simulink model "ster_cyfrowe"  (R2021b)
settings: Solver=VariableStepAuto  StartTime=0.0  StopTime=""  RelTol=1e-3
undefined symbols (not defined in the file or in its folder): kr, Td, Ti, Tp
settings Model: Creator=roman  LastModifiedBy=roman

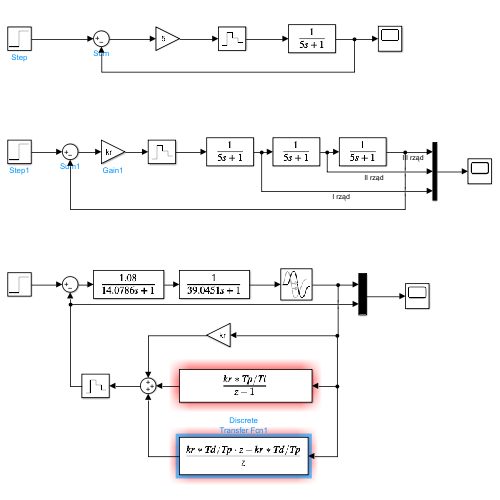
[thumbnail: Simulink's stored preview of the top-level diagram]
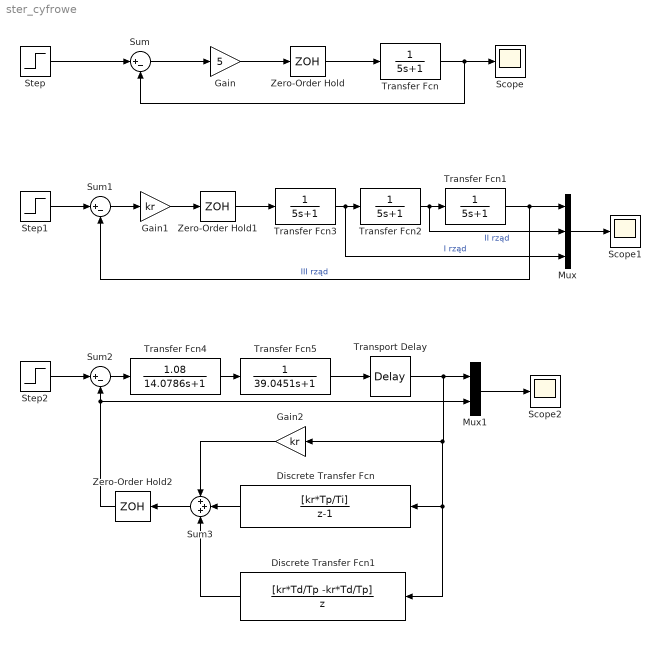
== system ster_cyfrowe ==
  Discrete Transfer Fcn : DiscreteTransferFcn  Numerator=[kr*Tp/Ti]  Denominator=[1 -1]
  Discrete Transfer Fcn1 : DiscreteTransferFcn  Numerator=[kr*Td/Tp -kr*Td/Tp]  Denominator=[1 0]  SampleTime=Tp
  Gain : Gain  Gain=5
  Gain1 : Gain  Gain=kr
  Gain2 : Gain  Gain=kr
  Mux : Mux  Inputs=3
  Mux1 : Mux  Inputs=2
  Scope : Scope
  Scope1 : Scope
  Scope2 : Scope
  Step : Step  SampleTime=Tp
  Step1 : Step  SampleTime=Tp
  Step2 : Step  SampleTime=Tp
  Sum : Sum  Inputs=|+-
  Sum1 : Sum  Inputs=|+-
  Sum2 : Sum  Inputs=|+-
  Sum3 : Sum  Inputs=+++
  Transfer Fcn{,1..3} (4 alike) : TransferFcn  Denominator=[5 1]
  Transfer Fcn4 : TransferFcn  Numerator=[1.08]  Denominator=[14.0786 1]
  Transfer Fcn5 : TransferFcn  Denominator=[39.0451 1]
  Transport Delay : TransportDelay  DelayTime=15.1975  PadeOrder=5
  Zero-Order Hold : ZeroOrderHold  SampleTime=Tp
  Zero-Order Hold1 : ZeroOrderHold  SampleTime=Tp
  Zero-Order Hold2 : ZeroOrderHold  SampleTime=Tp
  wires:
  Step/1 -> Sum/1
  Sum/1 -> Gain/1
  Gain/1 -> Zero-Order Hold/1
  Zero-Order Hold/1 -> Transfer Fcn/1
  Transfer Fcn/1 -> Scope/1, Sum/2
  Transfer Fcn3/1 -> Mux/3, Transfer Fcn2/1  "I rząd"
  Step1/1 -> Sum1/1
  Sum1/1 -> Gain1/1
  Transfer Fcn2/1 -> Mux/2, Transfer Fcn1/1  "II rząd"
  Mux/1 -> Scope1/1
  Transfer Fcn1/1 -> Mux/1, Sum1/2  "III rząd"
  Gain1/1 -> Zero-Order Hold1/1
  Zero-Order Hold1/1 -> Transfer Fcn3/1
  Transfer Fcn4/1 -> Transfer Fcn5/1
  Transfer Fcn5/1 -> Transport Delay/1
  Sum3/1 -> Zero-Order Hold2/1
  Zero-Order Hold2/1 -> Mux1/2, Sum2/2
  Step2/1 -> Sum2/1
  Sum2/1 -> Transfer Fcn4/1
  Mux1/1 -> Scope2/1
  Transport Delay/1 -> Discrete Transfer Fcn1/1, Discrete Transfer Fcn/1, Gain2/1, Mux1/1
  Discrete Transfer Fcn1/1 -> Sum3/3
  Discrete Transfer Fcn/1 -> Sum3/2
  Gain2/1 -> Sum3/1
